simulink model "test"  (R2014a)
settings: Solver=VariableStepDiscrete  StartTime=0.0  StopTime=10.0  RelTol=1e-3
undefined symbols (not defined in the file): fdesignblkfcn, gcbh
libraries: simulink x1, dspsrcs4 x1, fl_lib x1, commnoisgen2 x1
settings Model: Creator=zain  LastModifiedBy=zain

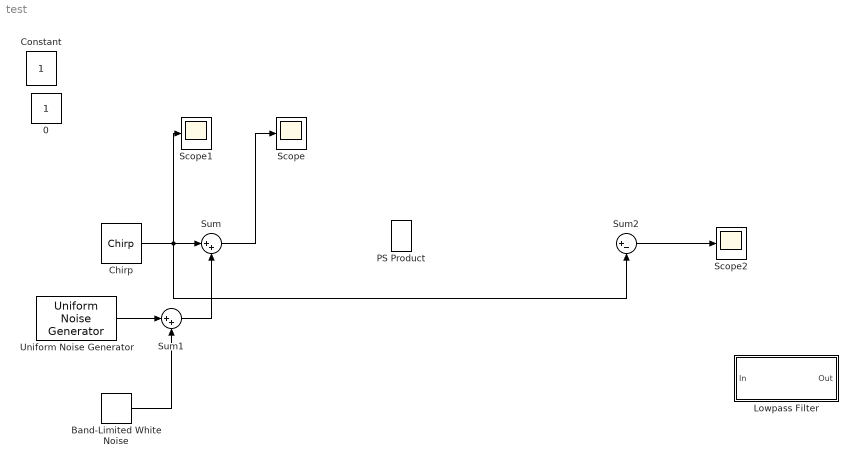
== system test ==
  Band-Limited White Noise : simulink/Sources/Band-Limited White Noise  Cov=[0.1]  Ts=0.1  seed=[23341]
  Chirp : dspsrcs4/Chirp  sweep=Linear  mode=Unidirectional  f0=1000  f1=4000  t1=1  Tsweep=2  phase=0  Ts=1/8000  spf=1  datatype=Double
  Lowpass Filter : Subsystem  DialogController=fdesignblkfcn  InitFcn=fdesignblkfcn(gcbh, {'InitFcn'});  mask(Lowpass Filter){}
      mask help: Design a lowpass filter
      settings: CopyFcn=fdesignblkfcn(gcbh, {'CopyFcn'});
      mask Help: helpview(mapfilelocation('dsp'), 'dsplowpassfilter');
      mask Display: disp('Lowpass')
  PS Product : fl_lib/Physical Signals/Functions/PS Product
  Scope : Scope
  Scope1 : Scope
  Scope2 : Scope
      settings: SaveName=ScopeData2
  Sum : Sum  Inputs=|++
  Sum1 : Sum  Inputs=|++
  Sum2 : Sum  Inputs=|+-
  Uniform Noise Generator : commnoisgen2/Uniform Noise Generator  low=0  up=1  seed=31  Ts=1  frameBased=off  sampPerFrame=1  orient=off  outDataType=double
  0 : Constant  IOType=siggen
  Constant : Constant  IOType=siggen  VectorParams1D=off  SampleTime=1
  wires:
  Chirp/1 -> Sum2/2, Scope1/1, Sum/1
  Uniform Noise Generator/1 -> Sum1/1
  Sum1/1 -> Sum/2
  Band-Limited White Noise/1 -> Sum1/2
  Sum/1 -> Scope/1
  ? -> ?
  ? -> Sum2/1
  Sum2/1 -> Scope2/1

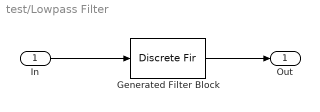
== system test/Lowpass Filter ==
  In : Inport
  Generated Filter Block : DiscreteFir  Tag=BlockMethodSubSystem  Coefficients=[-0.0024228738523269142 -0.002083244982079274 0.0067703446401187091 0.016731945423489058 0.011117076081077608 -0.0062311454141445394 -0.008401617186026911 0.0092567976151380175 0.012982883808855752 -0.010121234703278968 -0.018273518733782485 0.011431962071777957 0.02617588858040763 -0.012489027835322923 -0.037996623145463579 0.013388945199366963 0.058155465814729891 -0.014048043515808939 -0.10272466857882172 0.014462275771238358 0.31716649721769491 0.48538764678732504 0.31716649721769491 0.014462275771238358 -0.10272466857882172 -0.014048043515808939 0.058155465814729891 0.013388945199366963 -0.037996623145463579 -0.012489027835322923 0.02617588858040763 0.011431962071777957 -0.018273518733782485 -0.010121234703278968 0.012982883808855752 0.0092567976151380175 -0.008401617186026911 -0.0062311454141445394 0.011117076081077608 0.016731945423489058 0.0067703446401187091 -0.002083244982079274 -0.0024228738523269142]  InputProcessing=Columns as channels (frame based)
  Out : Outport
  wires:
  In/1 -> Generated Filter Block/1
  Generated Filter Block/1 -> Out/1
